simulink model "consumption_FrictionSimulation"  (R2021a)
settings: Solver=FixedStepAuto  StartTime=0.0  StopTime=3.0  FixedStep=1e-6  RelTol=1e-3
values from neighbouring files (symbols this model uses):
  duckWeight = 0.0708    [consumptionTorqueSimWS.mat]
  forcePeriod = 0.2    [consumptionTorqueSimWS.mat]
  forcePulseWidthPercent = 99    [consumptionTorqueSimWS.mat]
  momentArmLength = 0.0635    [consumptionTorqueSimWS.mat]
  phase0 = 0    [consumptionTorqueSimWS.mat]
  phase1 = 0    [consumptionTorqueSimWS.mat]
  phase2 = 0    [consumptionTorqueSimWS.mat]
settings Model: Creator=natha  LastModifiedBy=natha

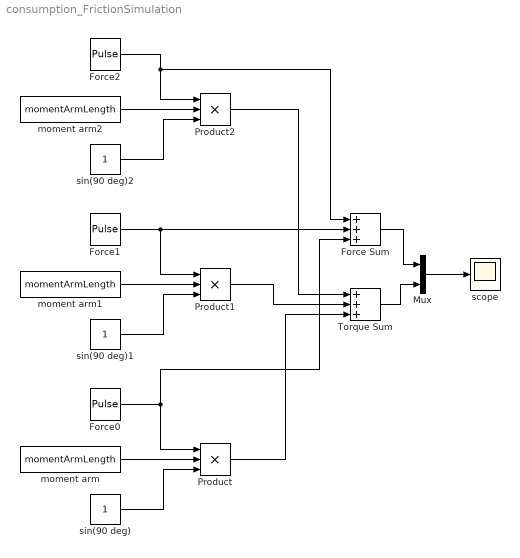
== system consumption_FrictionSimulation ==
  Force Sum : Sum  Inputs=+++
  Force0 : DiscretePulseGenerator  PulseType=Time based  Amplitude=9.8*duckWeight  Period=forcePeriod  PulseWidth=forcePulseWidthPercent  PhaseDelay=phase0
  Force1 : DiscretePulseGenerator  PulseType=Time based  Amplitude=9.8*duckWeight  Period=forcePeriod  PulseWidth=forcePulseWidthPercent  PhaseDelay=phase1
  Force2 : DiscretePulseGenerator  PulseType=Time based  Amplitude=9.8*duckWeight  Period=forcePeriod  PulseWidth=forcePulseWidthPercent  PhaseDelay=phase2
  Mux : Mux  Inputs=2
  Product : Product  Inputs=3
  Product1 : Product  Inputs=3
  Product2 : Product  Inputs=3
  Torque Sum : Sum  Inputs=+++
  moment arm : Constant  Value=momentArmLength
  moment arm1 : Constant  Value=momentArmLength
  moment arm2 : Constant  Value=momentArmLength
  scope : Scope
  sin(90 deg) : Constant
  sin(90 deg)1 : Constant
  sin(90 deg)2 : Constant
  wires:
  Product/1 -> Torque Sum/3
  sin(90 deg)/1 -> Product/3
  Force0/1 -> Force Sum/3, Product/1
  moment arm/1 -> Product/2
  Product1/1 -> Torque Sum/2
  sin(90 deg)1/1 -> Product1/3
  moment arm1/1 -> Product1/2
  Force1/1 -> Force Sum/2, Product1/1
  Product2/1 -> Torque Sum/1
  sin(90 deg)2/1 -> Product2/3
  moment arm2/1 -> Product2/2
  Force2/1 -> Force Sum/1, Product2/1
  Force Sum/1 -> Mux/1
  Torque Sum/1 -> Mux/2
  Mux/1 -> scope/1
